simulink model "TerminateFcn"  (R2022a)
settings: Solver=FixedStepAuto  StartTime=0.0  StopTime=Inf  FixedStep=SAMPLING_TIME  RelTol=1e-3
undefined symbols (not defined in the file): SAMPLING_TIME
Description:
  | % Copyright 2019 The MathWorks, Inc.
settings Model: DataDictionary=Parameters.sldd  EnableAccessToBaseWorkspace=off  Creator=sdupertu  LastModifiedBy=sebas
settings SolverCC: AlgebraicLoopSolver=TrustRegion
settings DataIOCC: SaveOutput=off  SaveTime=off
settings OptimizationCC: DefaultParameterBehavior=Inlined  EnhancedBackFolding=on  PassReuseOutputArgsAs=Individual arguments  OptimizeBlockOrder=speed  DifferentSizesBufferReuse=on  OptimizationCustomize=off  EfficientTunableParamExpr=on
settings DebuggingCC: ParameterTunabilityLossMsg=error  UnconnectedInputMsg=warning  UnconnectedOutputMsg=warning  UnconnectedLineMsg=warning  PregeneratedLibrarySubsystemCodeDiagnostic=none  SFMachineParentedDataDiag=warning  ArithmeticOperatorsInVariantConditions=warning
settings ModelReferenceCC: EnableParallelModelReferenceBuilds=on
settings SFSimCC: SimUseLocalCustomCode=off  MATLABDynamicMemAlloc=off  CustomCodeUndefinedFunction=UseInterfaceOnly
settings RTWCC: SystemTargetFile=ert.tlc  TemplateMakefile=ert_default_tmf  GenerateReport=on  RTWUseLocalCustomCode=off  IncludeHyperlinkInReport=on  LaunchReport=on  GenerateTraceInfo=on  GenerateTraceReport=on  GenerateTraceReportSl=on  GenerateTraceReportSf=on  GenerateTraceReportEml=on  GenerateWebview=on  GenerateCodeMetricsReport=on  DLArmComputeVersion=19.05
settings CodeAppCC: ForceParamTrailComments=on  IgnoreCustomStorageClasses=off  MaxIdLength=61  OperatorAnnotations=on  SimulinkDataObjDesc=on  SFDataObjDesc=on  InsertBlockDesc=on
settings ERTTargetCC: TargetLangStandard=C99 (ISO)  GenerateSampleERTMain=on  InlinedParameterPlacement=NonHierarchical  ERTCustomFileTemplate=example_file_process.tlc

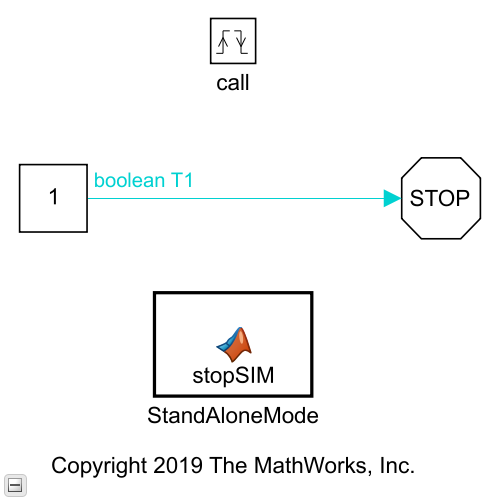
[thumbnail: Simulink's stored preview of the top-level diagram]
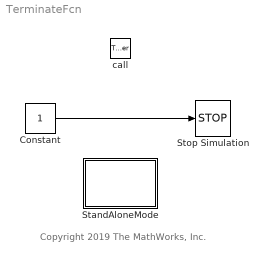
== system TerminateFcn ==
  note: Copyright 2019 The MathWorks, Inc.
  call : TriggerPort  TriggerType=either  VariantControl=Variant  PortDimensions=1  TriggerSignalSampleTime=[SAMPLING_TIME,0]
  Constant : Constant  OutDataTypeStr=boolean  SampleTime=-1
  StandAloneMode : MATLAB Function  TreatAsAtomicUnit=on
  Stop Simulation : Stop
  wires:
  Constant/1 -> Stop Simulation/1

== matlab function TerminateFcn/StandAloneMode ==
function stopSIM
  %#codegen
  if coder.target('Rtw')
  fprintf('The Master Switch of the Parking Meter Interface is switched off.\n');
  fprintf('Therefore the application has stopped and it can be closed.\n');
  % Include the header file containing the needed function declaration
  coder.cinclude('stdlib.h');
  % Stop the main standalone executable properly
  coder.ceval('exit',int32(0));
  end
end
